simulink model "inverse_kinematics"  (R2021a)
settings: Solver=VariableStepAuto  StartTime=0.0  StopTime=10.0  RelTol=1e-3
settings Model: Creator=kbhar  LastModifiedBy=kbhar

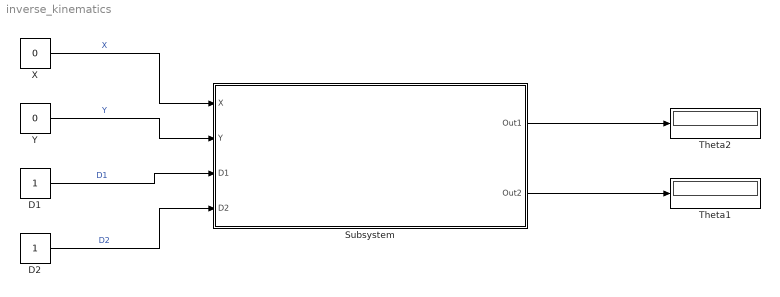
== system inverse_kinematics ==
  D1 : Constant
  D2 : Constant
  Subsystem : Subsystem
  Theta1 : Display
  Theta2 : Display
  X : Constant  Value=0
  Y : Constant  Value=0
  wires:
  X/1 -> Subsystem/1(X)  "X"
  Y/1 -> Subsystem/2(Y)  "Y"
  D1/1 -> Subsystem/3(D1)  "D1"
  D2/1 -> Subsystem/4(D2)  "D2"
  Subsystem/1(Out1) -> Theta2/1
  Subsystem/2(Out2) -> Theta1/1

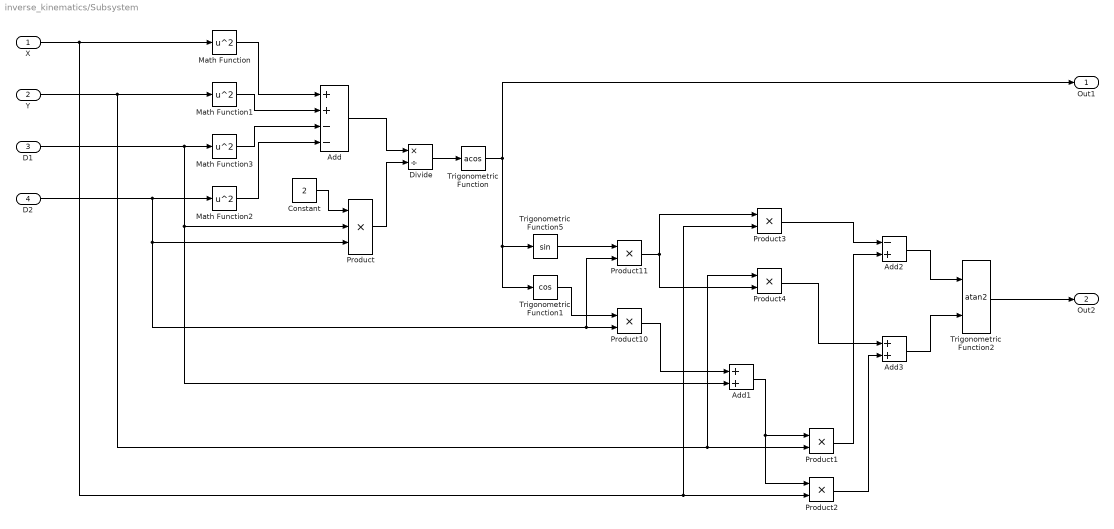
== system inverse_kinematics/Subsystem ==
  X : Inport
  Y : Inport  Port=2
  D1 : Inport  Port=3
  D2 : Inport  Port=4
  Add : Sum  Inputs=++--
  Add1 : Sum
  Add2 : Sum  Inputs=-+
  Add3 : Sum
  Constant : Constant  Value=2
  Divide : Product  Inputs=*/
  Math Function{,1..3} (4 alike) : Math  Operator=square  SaturateOnIntegerOverflow=on
  Product : Product  Inputs=3
  Product{1..4,10..11} (6 alike) : Product
  Trigonometric Function : Trigonometry  Operator=acos
  Trigonometric Function1 : Trigonometry  Operator=cos
  Trigonometric Function2 : Trigonometry  Operator=atan2
  Trigonometric Function5 : Trigonometry
  Out1 : Outport
  Out2 : Outport  Port=2
  wires:
  Trigonometric Function/1 -> Out1/1, Trigonometric Function1/1, Trigonometric Function5/1
  Trigonometric Function1/1 -> Product10/1
  D1/1 -> Add1/2, Product/2, Math Function3/1
  Math Function2/1 -> Add/4
  Trigonometric Function5/1 -> Product11/1
  X/1 -> Product2/2, Product3/2, Math Function/1
  Product/1 -> Divide/2
  Math Function3/1 -> Add/3
  Add/1 -> Divide/1
  Math Function1/1 -> Add/2
  Product2/1 -> Add3/2
  Product11/1 -> Product3/1, Product4/2
  Product1/1 -> Add2/2
  Add2/1 -> Trigonometric Function2/1
  Divide/1 -> Trigonometric Function/1
  Product3/1 -> Add2/1
  D2/1 -> Math Function2/1, Product11/2, Product10/2, Product/3
  Add1/1 -> Product1/1, Product2/1
  Math Function/1 -> Add/1
  Product10/1 -> Add1/1
  Product4/1 -> Add3/1
  Constant/1 -> Product/1
  Add3/1 -> Trigonometric Function2/2
  Y/1 -> Product1/2, Product4/1, Math Function1/1
  Trigonometric Function2/1 -> Out2/1
